simulink model "masacalcio"  (Simulink 7.5)
settings: Solver=ode45  StartTime=0.0  StopTime=10.0  RelTol=1e-3
settings Model: Creator=My Laptop  LastModifiedBy=My Laptop

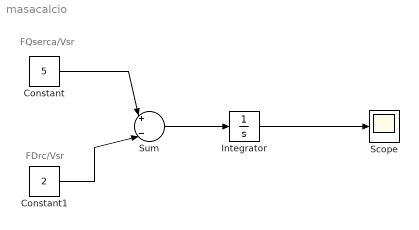
== system masacalcio ==
  note: FQserca/Vsr
  note: FDrc/Vsr
  Constant : Constant  Value=5  OutDataType=fixdt(1, 16)  OutScaling=2^0
  Constant1 : Constant  Value=2  OutDataType=fixdt(1, 16)  OutScaling=2^0
  Integrator : Integrator
  Scope : Scope
  Sum : Sum  Inputs=|+|-|  OutDataType=fixdt(1, 16)  OutScaling=2^0
  wires:
  Sum/1 -> Integrator/1
  Constant/1 -> Sum/1
  Constant1/1 -> Sum/2
  Integrator/1 -> Scope/1
